simulink model "mert_buses"  (Simulink 7.6)
settings: Solver=FixedStepDiscrete  SolverMode=SingleTasking  StartTime=0.0  StopTime=10  RelTol=1e-3
PostLoadFcn:
  | clear elems;
  | elems(1) = Simulink.BusElement;
  | elems(1).Name = 'a1';
  | elems(1).Dimensions = 4;
  | elems(1).DimensionsMode = 'Fixed';
  | elems(1).DataType = 'fixdt(0,16,4, ''DataTypeOverride'', ''Off'')';
  | elems(1).SampleTime = -1;
  | elems(1).Complexity = 'real';
  | elems(1).SamplingMode = 'Sample based';
  | 
  | BusObject = Simulink.Bus;
  | BusObject.HeaderFile = '';
  | BusObject.Description = sprintf('');
  | BusObject.Elements = elems;
  | assignin('base', 'BusObject', BusObject)
model workspace: external: MAT-File (data not in the file)
Description:
  | Algorithm Design
CloseFcn:
  | rtwprivate ssgencode ModelCloseRequest msig_init_values
settings Model: Creator=The MathWorks Inc.  LastModifiedBy=mkachmar  ParamWorkspaceSource=ReferencedWorkspace  CovMetricSettings=d  ExtModeTrigMode=oneshot  ExtModeArmWhenConnect=off  ExtModeAutoUpdateStatusClock=off
settings MATStruct: SampleTime=1  Offset=0  Priority=[41.0]
settings DataIOCC: ExternalInput=inputSeries__AnzX{1}, inputSeries__AnzX{2}  LimitDataPoints=off  SaveFormat=StructureWithTime  SaveOutput=off  SignalLogging=off  DSMLogging=off  SaveTime=off  SignalLoggingName=sigsOut
settings OptimizationCC: InlineParams=on  InlineInvariantSignals=on  StateBitsets=on  DataBitsets=on  UseTempVars=on  ZeroExternalMemoryAtStartup=off  ZeroInternalMemoryAtStartup=off  EfficientFloat2IntCast=on  EfficientMapNaN2IntZero=off  OptimizeModelRefInitCode=on  LifeSpan=1  BufferReusableBoundary=off
settings DebuggingCC: CheckExecutionContextPreStartOutputMsg=on  CheckExecutionContextRuntimeOutputMsg=on  SolverPrmCheckMsg=none  IntegerOverflowMsg=none  BusObjectLabelMismatch=error  RootOutportRequireBusObject=none  StrictBusMsg=ErrorOnBusTreatedAsVector
settings HardwareCC: ProdBitPerLong=64  ProdIntDivRoundTo=Zero  ProdEndianess=LittleEndian  ProdWordSize=64  ProdHWDeviceType=Specified  TargetHWDeviceType=Generic->32-bit Embedded Processor
settings ModelReferenceCC: UpdateModelReferenceTargets=IfOutOfDate
settings SFSimCC: SimParseCustomCode=off
settings RTWCC: SystemTargetFile=ert.tlc  TemplateMakefile=ert_default_tmf  Description=Real-Time Workshop Embedded Coder  ProcessScript=ert_make_rtw_hook  GenerateCodeInfo=on
settings CodeAppCC: ForceParamTrailComments=on  IgnoreCustomStorageClasses=off  InsertBlockDesc=on
settings ERTTargetCC: MultiwordLength=2048  GenerateSampleERTMain=on  InlinedParameterPlacement=NonHierarchical  ERTCustomFileTemplate=example_file_process.tlc  ConvertIfToSwitch=off

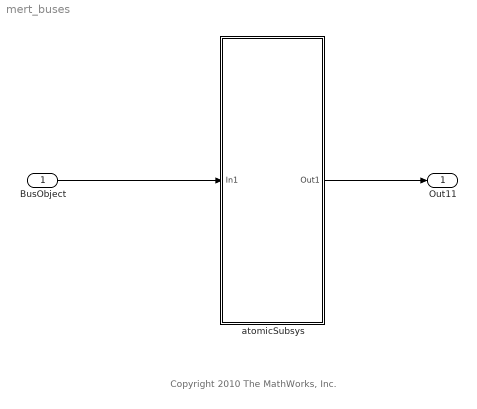
== system mert_buses ==
  note: Copyright 2010 The MathWorks, Inc.
  BusObject : Inport  OutDataTypeStr=Bus: BusObject  Interpolate=off  BusOutputAsStruct=on
  atomicSubsys : Subsystem  TreatAsAtomicUnit=on
  Out11 : Outport
  wires:
  BusObject/1 -> atomicSubsys/1(In1)
  atomicSubsys/1(Out1) -> Out11/1

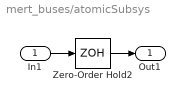
== system mert_buses/atomicSubsys ==
  In1 : Inport
  Zero-Order Hold2 : ZeroOrderHold  SampleTime=-1
  Out1 : Outport
  wires:
  In1/1 -> Zero-Order Hold2/1
  Zero-Order Hold2/1 -> Out1/1
